simulink model "jellystone"  (R2016b)
settings: Solver=FixedStepAuto  StartTime=0.0  StopTime=30  FixedStep=.1  RelTol=1e-3
undefined symbols (not defined in the file or in its folder): wolf
settings Model: Creator=thomaskennedy  LastModifiedBy=thomaskennedy

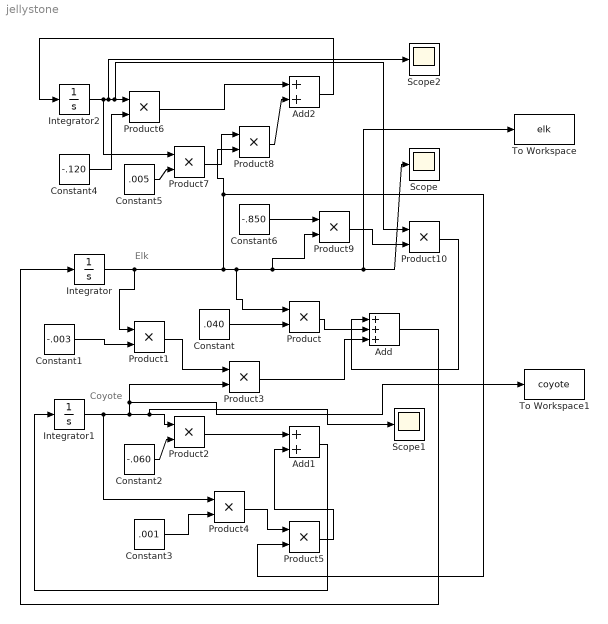
== system jellystone ==
  note: Elk
  note: Coyote
  Add : Sum  Inputs=+++
  Add1 : Sum
  Add2 : Sum
  Constant : Constant  Value=.040
  Constant1 : Constant  Value=-.003
  Constant2 : Constant  Value=-.060
  Constant3 : Constant  Value=.001
  Constant4 : Constant  Value=-.120
  Constant5 : Constant  Value=.005
  Constant6 : Constant  Value=-.850
  Integrator : Integrator  InitialCondition=31.217
  Integrator1 : Integrator  InitialCondition=2.017
  Integrator2 : Integrator  InitialCondition=wolf
  Product{,1..10} (11 alike) : Product
  Scope : Scope
  Scope1 : Scope
  Scope2 : Scope
  To Workspace : ToWorkspace  VariableName=elk  SampleTime=-1
  To Workspace1 : ToWorkspace  VariableName=coyote  SampleTime=-1
  wires:
  Constant/1 -> Product/2
  Product/1 -> Add/2
  Constant1/1 -> Product1/2
  Constant2/1 -> Product2/2
  Product1/1 -> Product3/1
  Product3/1 -> Add/3
  Product2/1 -> Add1/1
  Constant3/1 -> Product4/2
  Integrator/1 -> Product1/1, Product8/2, Product5/2, Product/1, Product9/2, To Workspace/1, Scope/1
  Product4/1 -> Product5/1
  Product5/1 -> Add1/2
  Add1/1 -> Integrator1/1
  Integrator1/1 -> Product4/1, To Workspace1/1, Product3/2, Scope1/1, Product2/1
  Constant4/1 -> Product6/2
  Product6/1 -> Add2/1
  Constant5/1 -> Product7/2
  Product7/1 -> Product8/1
  Product8/1 -> Add2/2
  Add2/1 -> Integrator2/1
  Constant6/1 -> Product9/1
  Product9/1 -> Product10/2
  Integrator2/1 -> Product7/1, Scope2/1, Product10/1, Product6/1
  Product10/1 -> Add/1
  Add/1 -> Integrator/1
